simulink subsystem "PieroModel"  (R2023b)
settings: Solver=VariableStepAuto  StartTime=0.0  StopTime=10.0  RelTol=1e-3
settings Model: Creator=Andrés  LastModifiedBy=Andrés

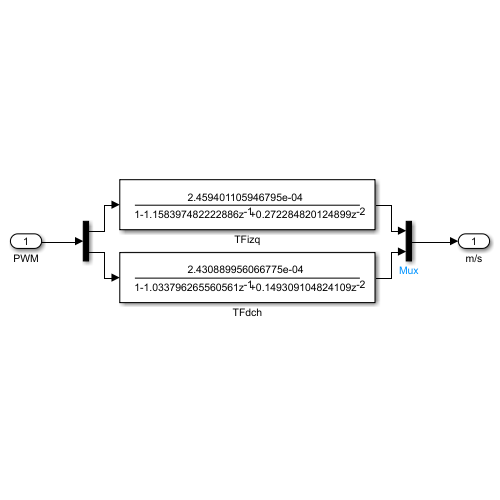
[thumbnail: Simulink's stored preview of the top-level diagram]
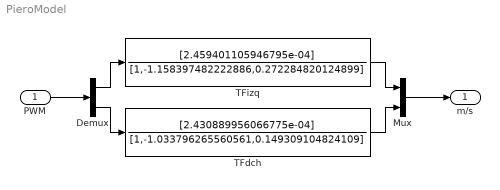
== system PieroModel ==
  PWM : Inport
  Demux : Demux  Outputs=2
  Mux : Mux  Inputs=2
  TFdch : DiscreteFilter  Numerator=[2.430889956066775e-04]  Denominator=[1,-1.033796265560561,0.149309104824109]
  TFizq : DiscreteFilter  Numerator=[2.459401105946795e-04]  Denominator=[1,-1.158397482222886,0.272284820124899]
  m/s : Outport
  wires:
  Mux/1 -> m/s/1
  PWM/1 -> Demux/1
  Demux/1 -> TFizq/1
  TFizq/1 -> Mux/1
  Demux/2 -> TFdch/1
  TFdch/1 -> Mux/2
